simulink model "Spacecraft_dynamics"  (R2023b)
settings: Solver=VariableStepAuto  StartTime=0.0  StopTime=10.0  RelTol=1e-3
settings Model: Creator=tiwan  LastModifiedBy=tiwan

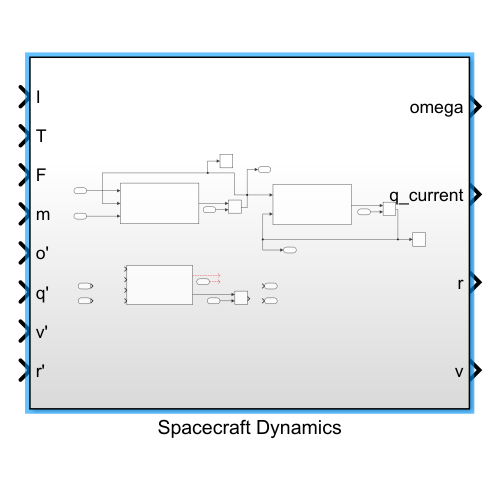
[thumbnail: Simulink's stored preview of the top-level diagram]
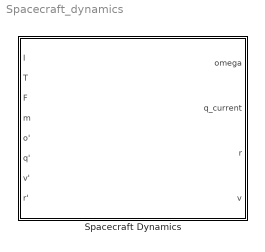
== system Spacecraft_dynamics ==
  Spacecraft Dynamics : Subsystem

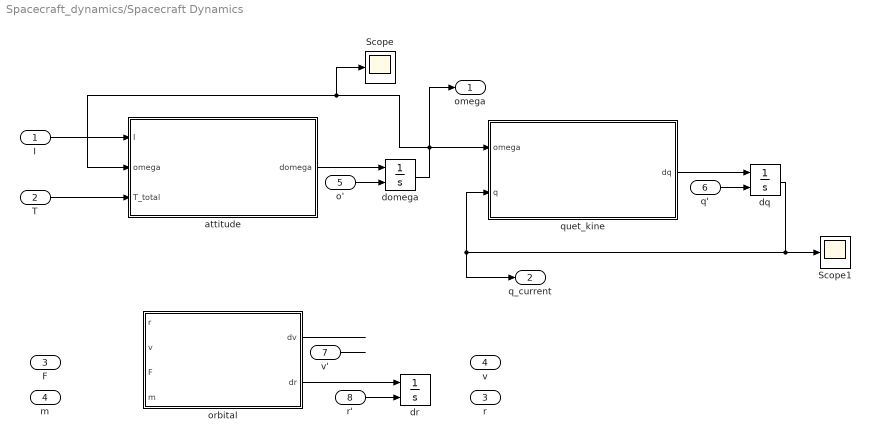
== system Spacecraft_dynamics/Spacecraft Dynamics ==
  I : Inport
  T : Inport  Port=2
  F : Inport  Port=3
  m : Inport  Port=4
  o' : Inport  Port=5
  q' : Inport  Port=6
  v' : Inport  Port=7
  r' : Inport  Port=8
  Scope : Scope
  Scope1 : Scope
  attitude : MATLAB Function  TreatAsAtomicUnit=on
  domega : Integrator  InitialConditionSource=external
  dq : Integrator  InitialConditionSource=external
  dr : Integrator  InitialConditionSource=external
  orbital : MATLAB Function  TreatAsAtomicUnit=on
  quet_kine : MATLAB Function  TreatAsAtomicUnit=on
  omega : Outport
  q_current : Outport  Port=2
  r : Outport  Port=3
  v : Outport  Port=4
  wires:
  attitude/1(domega) -> domega/1
  domega/1 -> omega/1, Scope/1, attitude/2(omega), quet_kine/1(omega)
  quet_kine/1(dq) -> dq/1
  dq/1 -> Scope1/1, quet_kine/2(q), q_current/1
  orbital/1(dv) -> ?
  orbital/2(dr) -> dr/1
  I/1 -> attitude/1(I)
  T/1 -> attitude/3(T_total)
  o'/1 -> domega/2
  q'/1 -> dq/2
  v'/1 -> ?
  r'/1 -> dr/2

== matlab function Spacecraft_dynamics/Spacecraft Dynamics/attitude ==
  data: I input; domega output; omega input; T_total input
function domega = angular_dynamics(I, omega, T_total)
% Safety checks
if any(isnan(omega)) || any(isinf(omega))
    omega = [0;0;0];
end
if any(isnan(T_total)) || any(isinf(T_total))
    T_total = [0;0;0];
end

omega_cross = [  0        -omega(3)  omega(2);
              omega(3)     0       -omega(1);
             -omega(2)  omega(1)     0    ];

% Prevent singular matrix issues
if det(I) < 1e-6
    I = I + 1e-3 * eye(3);  % Regularize inertia
end

domega = I \ (T_total - omega_cross * (I * omega));
end

== matlab function Spacecraft_dynamics/Spacecraft Dynamics/quet_kine ==
  data: omega input; dq output; q input
function dq = quaternion_kinematics(omega, q)
% omega: angular velocity [3x1]
% q: current quaternion [4x1]

Omega = [0       -omega(1) -omega(2) -omega(3);
         omega(1)  0        omega(3) -omega(2);
         omega(2) -omega(3) 0         omega(1);
         omega(3) omega(2) -omega(1)  0];

dq = 0.5 * Omega * q;
end

== matlab function Spacecraft_dynamics/Spacecraft Dynamics/orbital ==
  data: r input; dv output; v input; F input; m input; dr output
function [dv, dr] = orbital_dynamics(r, v, F, m)
% r: position vector [3x1]
% v: velocity vector [3x1]
% F: total force applied [3x1]
% m: spacecraft mass (scalar)

mu = 398600.4418;  % Earth's gravitational parameter, km^3/s^2

% Two-body gravity + applied force
r_norm = norm(r);
a_gravity = -mu * r / r_norm^3;
a_applied = F / m;

dv = a_gravity + a_applied;
dr = v;
end
